simulink model "WorkingFile"  (R2021a)
settings: Solver=FixedStepAuto  StartTime=0.0  StopTime=inf  FixedStep=1/100  RelTol=1e-3
settings Model: EnablePacing=on  PacingRate=25  Creator=Peska  LastModifiedBy=Peska

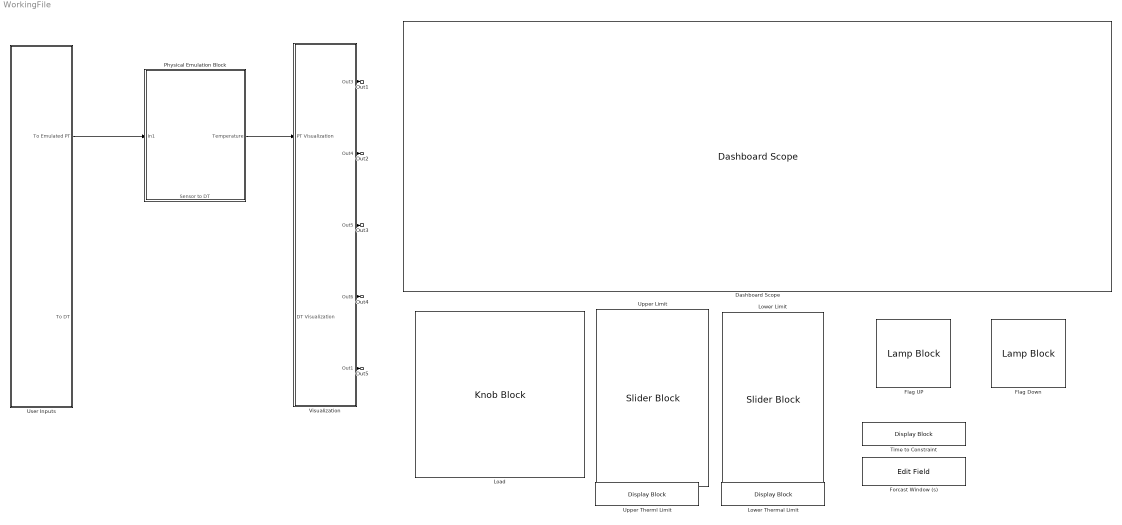
== system WorkingFile ==
  " Time to Constraint" : DisplayBlock  LabelPosition=Hide  Format=short  Transparency=1
  Dashboard Scope : DashboardScope  TimeSpan=50  Ymin=22  Ymax=27  UpdateMode=Scroll
  Flag Down : LampBlock  LabelPosition=Hide
  Flag UP : LampBlock  LabelPosition=Hide
  Forcast Window (s) : EditField  LabelPosition=Hide  ShowInitialText=on  Alignment=Center
  Load : KnobBlock  LabelPosition=Hide  ScaleMin=0.1  ScaleMax=7  TickInterval=1
  Lower Limit : SliderBlock  LabelPosition=Hide  ScaleMin=20  ScaleMax=80  TickInterval=10
  Lower Thermal Limit : DisplayBlock  LabelPosition=Hide  Format=shortG  Transparency=1
  Physical Emulation Block : Subsystem
      settings: PortSchema="{\"entries\":[{\"content\":{\"sides\":[{\"content\":{\"connectorIds\":[\"In1\"]},\"type\":\"ConnectorPlacement.EquallySpacedRectSide\",\"uuid\":\"8560139e-4285-4401-a1f9-6e73b4801051\"},{\"content\":{\"connectorIds\":[\"Out1\"],\"side\":\"RIGHT\"},\"type\":\"ConnectorPlacement.EquallySpacedRectSide\",\"uuid\":\"0f67ff7b-1654-419c-a011-ac6310eed1b7\"},{\"content\":{\"connectorIds\":[],\"side\":\"TOP\"},\"type\":\"ConnectorPlacement.EquallySpacedRectSide\",\"uuid\":\"736bff96-f03d-4d50-97ff-1700a1313303\"},{\"content\":{\"connectorIds\":[\"Out2\"],\"side\":\"BOTTOM\"},\"type\":\"ConnectorPlacement.EquallySpacedRectSide\",\"uuid\":\"ea04bb7b-7a64-4cd8-b38c-8dbcf65d1b9b\"}]},\"type\":\"ConnectorPlacement.EquallySpacedConnector\",\"uuid\":\"445e340e-037d-485f-9910-d1ac0550edc0\"}],\"packageUris\":[\"http://schema.mathworks.com/mf0/Connector/R2020b\"],\"version\":\"1.0\"}"
  Upper Limit : SliderBlock  LabelPosition=Hide  ScaleMin=20  ScaleMax=80  TickInterval=10
  Upper Therml Limit : DisplayBlock  LabelPosition=Hide  Format=shortG  Transparency=1
  User Inputs : Subsystem
  Visualization : Subsystem
  Out1 : Outport
  Out2 : Outport  Port=2
  Out3 : Outport  Port=3
  Out4 : Outport  Port=4
  Out5 : Outport  Port=5
  wires:
  Visualization/1(Out3) -> Out1/1
  Visualization/2(Out4) -> Out2/1
  Visualization/3(Out5) -> Out3/1
  Visualization/4(Out6) -> Out4/1
  Visualization/5(Out1) -> Out5/1
  User Inputs/1(To Emulated PT) -> Physical Emulation Block/1(In1)
  Physical Emulation Block/1(Temperature) -> Visualization/1("PT Visualization ")

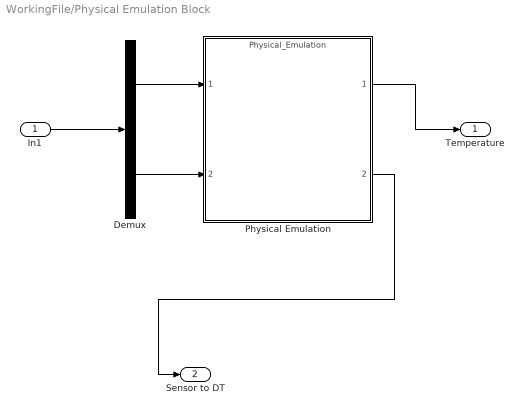
== system WorkingFile/Physical Emulation Block ==
  In1 : Inport
  Demux : Demux  Outputs=2
  Physical Emulation : ModelReference  ModelNameDialog=Physical_Emulation.slxp  ModelReferenceVersion=1.6  CopyOfModelProtected=on
  Temperature : Outport
  Sensor to DT : Outport  Port=2
  wires:
  Demux/1 -> Physical Emulation/1
  Demux/2 -> Physical Emulation/2
  Physical Emulation/2 -> Sensor to DT/1
  In1/1 -> Demux/1
  Physical Emulation/1 -> Temperature/1

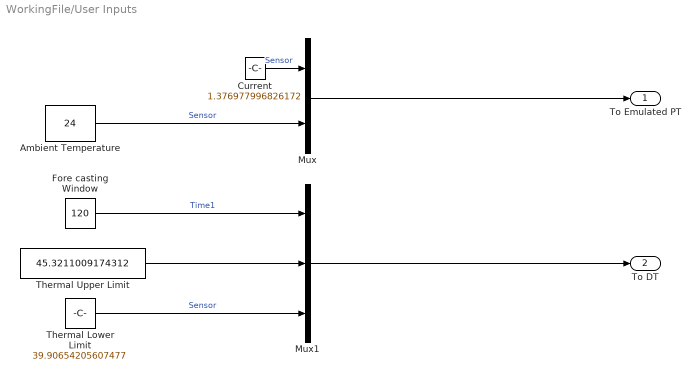
== system WorkingFile/User Inputs ==
  Ambient Temperature : Constant  Value=24
  Current : Constant  Value=1.376977996826172
  Fore casting Window : Constant  Value=120
  Mux : Mux  Inputs=2
  Mux1 : Mux  Inputs=3
  Thermal Lower Limit : Constant  Value=39.90654205607477
  Thermal Upper Limit : Constant  Value=45.3211009174312
  To Emulated PT : Outport
  To DT : Outport  Port=2
  wires:
  Fore casting Window/1 -> Mux1/1  "Time1"
  Thermal Upper Limit/1 -> Mux1/2
  Thermal Lower Limit/1 -> Mux1/3  "Sensor"
  Mux1/1 -> To DT/1
  Current/1 -> Mux/1  "Sensor"
  Ambient Temperature/1 -> Mux/2  "Sensor"
  Mux/1 -> To Emulated PT/1

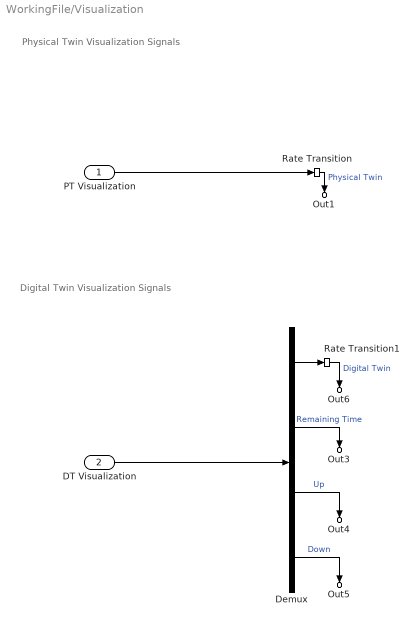
== system WorkingFile/Visualization ==
  note: Digital Twin Visualization Signals
  note: Physical Twin Visualization Signals
  "PT Visualization " : Inport
  DT Visualization : Inport  Port=2
  Demux : Demux
  Rate Transition : RateTransition  OutPortSampleTime=1
  Rate Transition1 : RateTransition  OutPortSampleTime=1
  Out3 : Outport
  Out4 : Outport  Port=2
  Out5 : Outport  Port=3
  Out6 : Outport  Port=4
  Out1 : Outport  Port=5
  wires:
  Demux/3 -> Out4/1  "Up"
  Rate Transition1/1 -> Out6/1  "Digital Twin"
  Demux/2 -> Out3/1  "Remaining Time"
  Demux/4 -> Out5/1  "Down"
  DT Visualization/1 -> Demux/1
  Demux/1 -> Rate Transition1/1
  Rate Transition/1 -> Out1/1  "Physical Twin"
  "PT Visualization "/1 -> Rate Transition/1
